simulink model "simulacija_regulacije"  (R2015b)
settings: Solver=VariableStepAuto  StartTime=0.0  StopTime=1000  MaxStep=0.01  RelTol=1e-3
undefined symbols (not defined in the file): Kh, Kz, Th, Tz
settings Model: Creator=Korisnik  LastModifiedBy=Korisnik

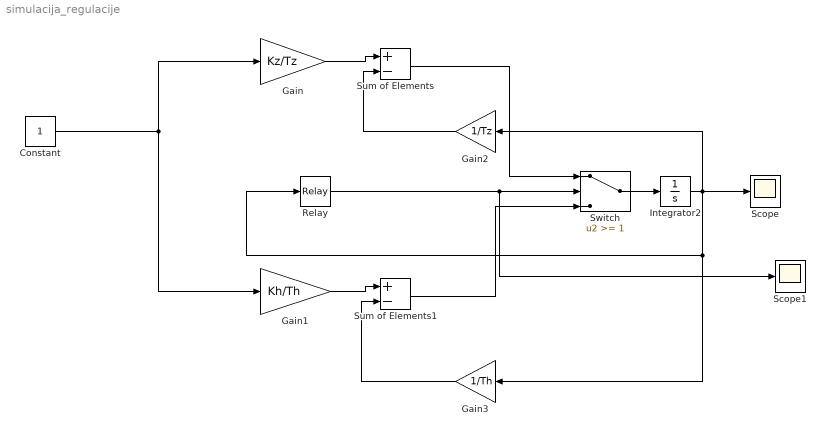
== system simulacija_regulacije ==
  Constant : Constant
  Gain : Gain  Gain=Kz/Tz
  Gain1 : Gain  Gain=Kh/Th
  Gain2 : Gain  Gain=1/Tz
  Gain3 : Gain  Gain=1/Th
  Integrator2 : Integrator
  Relay : Relay  OnSwitchValue=47.5  OffSwitchValue=44.5  OnOutputValue=0  OffOutputValue=1
  Scope : Scope
  Scope1 : Scope
  Sum of Elements : Sum  Inputs=+-
  Sum of Elements1 : Sum  Inputs=+-
  Switch : Switch  Threshold=1
  wires:
  Constant/1 -> Gain/1, Gain1/1
  Gain/1 -> Sum of Elements/1
  Gain1/1 -> Sum of Elements1/1
  Gain2/1 -> Sum of Elements/2
  Sum of Elements/1 -> Switch/1
  Gain3/1 -> Sum of Elements1/2
  Sum of Elements1/1 -> Switch/3
  Relay/1 -> Scope1/1, Switch/2
  Switch/1 -> Integrator2/1
  Integrator2/1 -> Gain2/1, Scope/1, Gain3/1, Relay/1
